simulink model "angle"  (R2024a)
settings: Solver=ode1  StartTime=0.0  StopTime=inf  FixedStep=0.01  RelTol=1e-3  EnableMultiTasking=on
libraries: arduinolib x4, slpidlib x1, arduinosensorlib x1, simulink_extras x1
settings Model: ExtModeTrigDuration=2  Creator=abane  LastModifiedBy=abane
settings SolverCC: AutoInsertRateTranBlk=on
settings OptimizationCC: EnhancedBackFolding=on  PassReuseOutputArgsAs=Individual arguments  ZeroExternalMemoryAtStartup=off  ZeroInternalMemoryAtStartup=off  MaxStackSize=64  OptimizeBlockOrder=speed  DifferentSizesBufferReuse=on  OptimizationCustomize=off  EfficientTunableParamExpr=on
settings DebuggingCC: ParameterTunabilityLossMsg=error
settings HardwareCC: ProdBitPerInt=16  ProdBitPerPointer=16  ProdBitPerSizeT=16  ProdBitPerPtrDiffT=16  ProdLargestAtomicFloat=None  ProdWordSize=8  ProdHWDeviceType=Atmel->AVR  UseEmbeddedCoderFeatures=off  UseSimulinkCoderFeatures=off
settings SFSimCC: MATLABDynamicMemAlloc=off
settings RTWCC: Description=Embedded Coder  SystemTargetFile=ert.tlc  HardwareBoard=Arduino Mega 2560  TemplateMakefile=ert_default_tmf  Toolchain=Arduino AVR  BuildConfiguration=Faster Runs
settings CodeAppCC: ForceParamTrailComments=on  IgnoreCustomStorageClasses=off  OperatorAnnotations=on  SimulinkDataObjDesc=on  SFDataObjDesc=on  InsertBlockDesc=on
settings ERTTargetCC: SupportContinuousTime=on  SupportNonInlinedSFcns=on  SupportVariableSizeSignals=on  ExtModeTransport=3  ExtModeStaticAlloc=on  ExtModeAutomaticAllocSize=off  ExtModeStaticAllocSize=2048  ExtModeMexFile=ext_xcp  ExtModeIntrfLevel=Level2 - Open

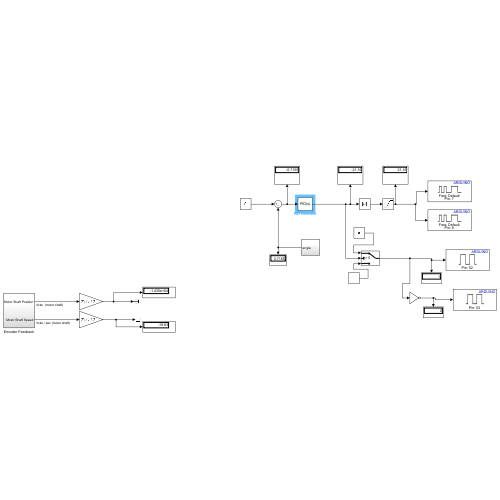
[thumbnail: Simulink's stored preview of the top-level diagram]
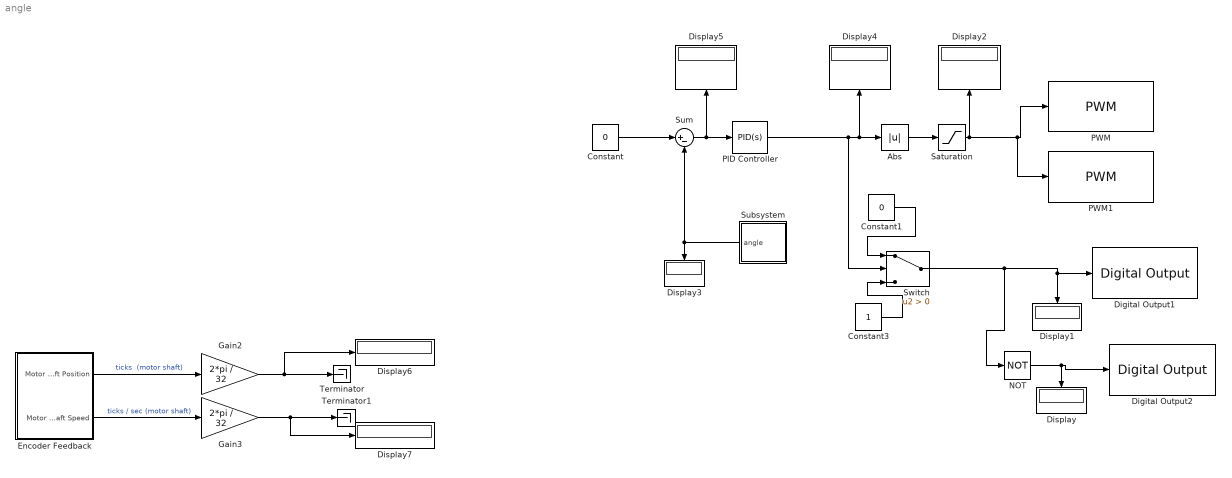
== system angle ==
  Abs : Abs  SaturateOnIntegerOverflow=off
  Constant : Constant  Value=0
  Constant1 : Constant  Value=0
  Constant3 : Constant
  Digital Output1 : arduinolib/Digital Output  pinNumber=52  Direction=output  blockPlatform=arduino
  Digital Output2 : arduinolib/Digital Output  pinNumber=53  Direction=output  blockPlatform=arduino
  Display{,1..7} (8 alike) : Display
  Encoder Feedback : Subsystem
  Gain2 : Gain  Gain=2*pi / 32
  Gain3 : Gain  Gain=2*pi / 32
  NOT : Logic  Operator=NOT  IconShape=distinctive  AllPortsSameDT=off  OutDataTypeStr=boolean
  PID Controller : slpidlib/PID Controller  Controller=PID  Form=Parallel  TimeDomain=Continuous-time  UseExternalTs=off  SampleTime=-1  IntegratorMethod=Forward Euler  FilterMethod=Forward Euler  ControllerParametersSource=internal  P=25  I=10  UseKiTs=off  D=0  UseExternalDerivativeSource=off  N=100  UseFilter=on  TunerSelectOption=Transfer Function Based (PID Tuner App)  InitialConditionSource=internal  InitialConditionForIntegrator=0  InitialConditionForFilter=0  DifferentiatorICPrevScaledInput=0  ExternalReset=none  TrackingMode=off  Kt=1  LimitOutput=off  SatLimitsSource=internal  UpperSaturationLimit=inf  LowerSaturationLimit=-inf  LinearizeAsGain=on  AntiWindupMode=none  Kb=1  LimitIntegrator=off  UpperIntegratorSaturationLimit=inf  LowerIntegratorSaturationLimit=-inf  POutMin=[]  POutMax=[]  IOutMin=[]  IOutMax=[]  DOutMin=[]  DOutMax=[]  NOutMin=[]  NOutMax=[]  SumOutMin=[]  SumOutMax=[]  SaturationOutMin=[]  SaturationOutMax=[]  PParamMin=[]  PParamMax=[]  IParamMin=[]  IParamMax=[]  DParamMin=[]  DParamMax=[]  NParamMin=[]  NParamMax=[]  KbParamMin=[]  KbParamMax=[]  KtParamMin=[]  KtParamMax=[]  KbOutMin=[]  KbOutMax=[]  KtOutMin=[]  KtOutMax=[]  IntegratorOutMin=[]  IntegratorOutMax=[]  FilterOutMin=[]  FilterOutMax=[]  SumI1OutMin=[]  SumI1OutMax=[]  SumI2OutMin=[]  SumI2OutMax=[]  SumI3OutMin=[]  SumI3OutMax=[]  SumI4OutMin=[]  SumI4OutMax=[]  SumDOutMin=[]  SumDOutMax=[]  DifferentiatorOutMin=[]  DifferentiatorOutMax=[]  FilterDiffOutCoefMin=[]  FilterDiffOutCoefMax=[]  ReciprocalOutMin=[]  ReciprocalOutMax=[]  SumDenOutMin=[]  SumDenOutMax=[]  SumNumOutMin=[]  SumNumOutMax=[]  DivideOutMin=[]  DivideOutMax=[]  UdiffTsProdOutMin=[]  UdiffTsProdOutMax=[]  NTsProdOutMin=[]  NTsProdOutMax=[]  UintegralTsProdOutMin=[]  UintegralTsProdOutMax=[]  UngainTsProdOutMin=[]  UngainTsProdOutMax=[]  ClampingZeroOutDataTypeStr=Inherit: Inherit via back propagation  ClampingZeroOutMin=[]  ClampingZeroOutMax=[]  FilterDenConstantOutDataTypeStr=Inherit: Inherit via back propagation  FilterDenConstantOutMin=[]  FilterDenConstantOutMax=[]  PCopyOutDataTypeStr=Inherit: Inherit via back propagation  PCopyOutMin=[]  PCopyOutMax=[]  NCopyOutDataTypeStr=Inherit: Inherit via back propagation  NCopyOutMin=[]  NCopyOutMax=[]  IntegratorContinuousStateAttributes=''  IntegratorStateMustResolveToSignalObject=off  IntegratorRTWStateStorageClass=Auto  FilterContinuousStateAttributes=''  FilterStateMustResolveToSignalObject=off  FilterRTWStateStorageClass=Auto  ParallelPVariant=InternalParameters  IdealPVariant=Disabled  IVariant=InternalParameters  DVariant=InternalParameters  IntegratorVariant=Continuous  SatVariant=Disabled  AWVariant=Passthrough  PCopyVariant=Disabled  TRVariant=Disabled  FdbkBlocksVariant=Forward  IdealPFdbkVariant=Disabled  SatFdbkVariant=Disabled  DerivativeFilterVariant=ContFilter  NVariant=InternalParameters  NCopyVariant=Disabled  FilterICVariant=InternalICsFilter  IntegratorICVariant=InternalICs  ExternalResetVariant=Disabled  TRSumVariant=Passthrough  SumFdbkVariant=Disabled  SumVariant=Sum_PID  TsampFilterVariant=InternalTs  TsampNgainVariant=Passthrough  TsampIntegralVariant=Disabled_SignalSpec  ExternalSaturationOutDataTypeStr=Inherit: Same as second input  DerivativeSourceVariant=ErrorSignal
  PWM : arduinolib/PWM  pinNumber=7  frequencyType=Default  desiredFrequency=490.2  achievableFrequency=490.2
  PWM1 : arduinolib/PWM  pinNumber=8  frequencyType=Default  desiredFrequency=490.2  achievableFrequency=490.2
  Saturation : Saturate  UpperLimit=255  LowerLimit=0
  Subsystem : Subsystem
  Sum : Sum  Inputs=|+-
  Switch : Switch  Criteria=u2 > Threshold  SaturateOnIntegerOverflow=off  InputSameDT=off
  Terminator : Terminator
  Terminator1 : Terminator
  wires:
  Sum/1 -> PID Controller/1, Display5/1
  Saturation/1 -> PWM1/1, PWM/1, Display2/1
  Subsystem/1(angle) -> Display3/1, Sum/2
  Constant/1 -> Sum/1
  Constant1/1 -> Switch/1
  Constant3/1 -> Switch/3
  Switch/1 -> NOT/1, Digital Output1/1, Display1/1
  PID Controller/1 -> Display4/1, Abs/1, Switch/2
  NOT/1 -> Digital Output2/1, Display/1
  Abs/1 -> Saturation/1
  Encoder Feedback/2(Motor Shaft Speed) -> Gain3/1  "ticks / sec (motor shaft)"
  Gain3/1 -> Display7/1, Terminator1/1
  Encoder Feedback/1(Motor Shaft Position) -> Gain2/1  "ticks  (motor shaft)"
  Gain2/1 -> Display6/1, Terminator/1

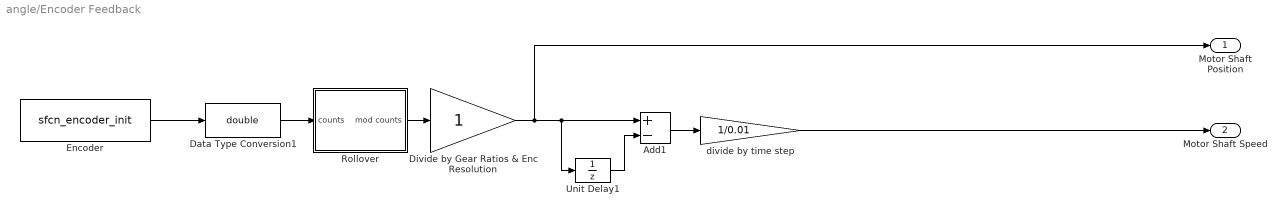
== system angle/Encoder Feedback ==
  Add1 : Sum  Inputs=+-
  Data Type Conversion1 : DataTypeConversion  OutDataTypeStr=double  SaturateOnIntegerOverflow=off  RndMeth=Floor
  Divide by Gear Ratios & Enc Resolution : Gain
  Encoder : S-Function  InitFcn=try, set_param(gcb,'FunctionName','sfcn_encoder_init'), end  FunctionName=sfcn_encoder_init  Parameters=uint8(0),uint8(3),uint8(1)  SFunctionModules=sfcn_encoder_init_wrapper.c  SFunctionDeploymentMode=off  EnableBusSupport=off  mask(S-Function Builder){}
      mask init:
      | val = [[.9  0.75 0.75 1 1 .9 .9 1]',[1 1 0.75 0.75 .9 .9 1 .9]'];try , sys = get_param(gcb,'SfunBuilderFcnName');if isempty(sys), sys = get_param(gcb,'FunctionName'); end,catch, sys = get_param(gcb,'FunctionName'); end
      settings: CopyFcn=set_param(gcbh,'LinkStatus','none')  PreSaveFcn=try, set_param(gcb,'FunctionName','sfcn_encoder_init'), end  OpenFcn=sfunctionwizard(gcbh)
      mask Display: plot(val(:,1),val(:,2)),disp(sys), port_label('output',1,'pos')
  Rollover : Subsystem
  Unit Delay1 : UnitDelay  SampleTime=-1  HasFrameUpgradeWarning=on
  divide by time step : Gain  Gain=1/0.01
  Motor Shaft Position : Outport
  Motor Shaft Speed : Outport  Port=2
  wires:
  Encoder/1 -> Data Type Conversion1/1
  Unit Delay1/1 -> Add1/2
  Data Type Conversion1/1 -> Rollover/1(counts)
  divide by time step/1 -> Motor Shaft Speed/1
  Add1/1 -> divide by time step/1
  Rollover/1(" mod counts") -> Divide by Gear Ratios & Enc Resolution/1
  Divide by Gear Ratios & Enc Resolution/1 -> Motor Shaft Position/1, Add1/1, Unit Delay1/1

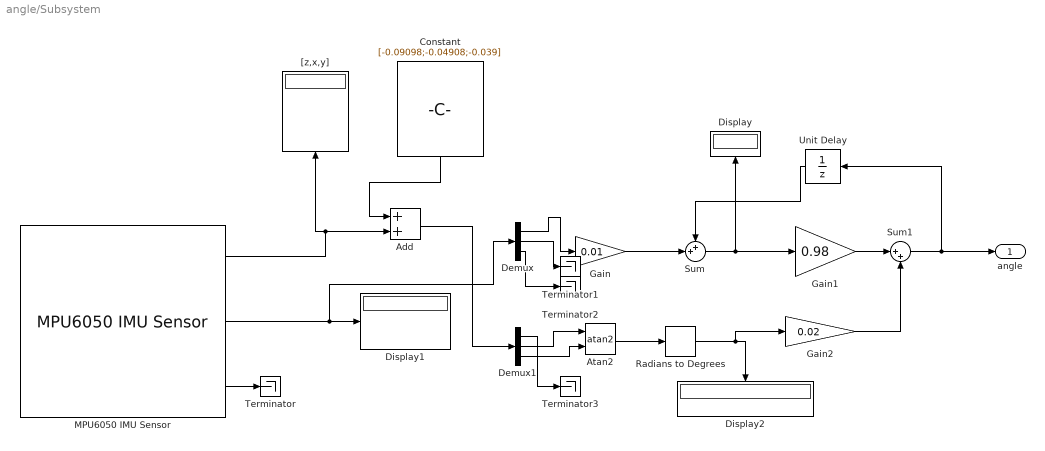
== system angle/Subsystem ==
  Add : Sum
  Atan2 : Trigonometry  Operator=atan2
  Constant : Constant  Value=[-0.09098;-0.04908;-0.039]  VectorParams1D=off
  Demux : Demux  Outputs=3
  Demux1 : Demux  Outputs=3
  Display : Display
  Display1 : Display
  Display2 : Display
  Gain : Gain  Gain=0.01
  Gain1 : Gain  Gain=0.98
  Gain2 : Gain  Gain=0.02
  MPU6050 IMU Sensor : arduinosensorlib/MPU6050 IMU Sensor  I2CModule=0  SlaveAddress=0x68  Accel=on  AngularRate=on  Temperature=off  Status=on  Timestamp=off  EulerAngles=off  Quat=off  AccelRange=2G  GyroRange=250 dps  DmpOdr=200 Hz  Dlpf=Accelerometer: 184Hz, Gyroscope: 188Hz  spf=1  SampleTime=-1  QueueSizeFactor=1
  Radians to Degrees : simulink_extras/Transformations/Radians to Degrees
  Sum : Sum  Inputs=++|
  Sum1 : Sum  Inputs=|++
  Terminator{,1..3} (4 alike) : Terminator
  Unit Delay : UnitDelay  SampleTime=-1  HasFrameUpgradeWarning=on
  "[z,x,y]" : Display
  angle : Outport
  wires:
  MPU6050 IMU Sensor/1 -> Add/2, "[z,x,y]"/1
  Demux1/1 -> Terminator3/1
  Sum/1 -> Gain1/1, Display/1
  MPU6050 IMU Sensor/2 -> Demux/1, Display1/1
  Gain/1 -> Sum/2
  Add/1 -> Demux1/1
  Constant/1 -> Add/1
  Atan2/1 -> Radians to Degrees/1
  Gain1/1 -> Sum1/1
  Demux/3 -> Terminator2/1
  Demux1/2 -> Atan2/1
  Demux1/3 -> Atan2/2
  Gain2/1 -> Sum1/2
  Radians to Degrees/1 -> Gain2/1, Display2/1
  MPU6050 IMU Sensor/3 -> Terminator/1
  Sum1/1 -> angle/1, Unit Delay/1
  Demux/1 -> Gain/1
  Unit Delay/1 -> Sum/1
  Demux/2 -> Terminator1/1

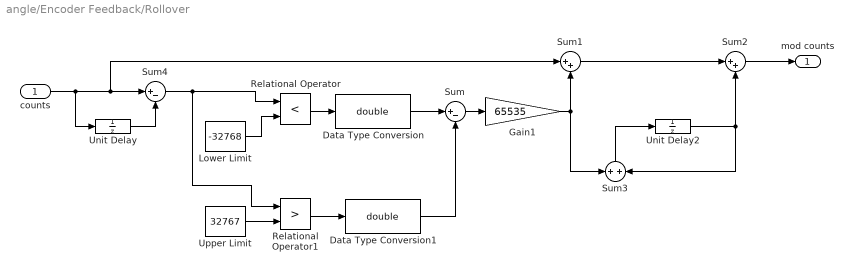
== system angle/Encoder Feedback/Rollover ==
  counts : Inport
  " Lower Limit" : Constant  Value=-32768
  " Upper Limit" : Constant  Value=32767
  Data Type Conversion : DataTypeConversion  OutDataTypeStr=double  SaturateOnIntegerOverflow=off
  Data Type Conversion1 : DataTypeConversion  OutDataTypeStr=double  SaturateOnIntegerOverflow=off
  Gain1 : Gain  Gain=65535
  Relational Operator : RelationalOperator  Operator=<  OutDataTypeStr=boolean  InputSameDT=off
  Relational Operator1 : RelationalOperator  Operator=>  OutDataTypeStr=boolean  InputSameDT=off
  Sum : Sum  Inputs=|+-
  Sum1 : Sum  Inputs=|++  OutDataTypeStr=double
  Sum2 : Sum  Inputs=|++
  Sum3 : Sum
  Sum4 : Sum  Inputs=|+-
  Unit Delay : UnitDelay  SampleTime=-1  HasFrameUpgradeWarning=on
  Unit Delay2 : UnitDelay  SampleTime=-1  HasFrameUpgradeWarning=on
  " mod counts" : Outport
  wires:
  counts/1 -> Unit Delay/1, Sum1/1, Sum4/1
  Sum2/1 -> " mod counts"/1
  Unit Delay/1 -> Sum4/2
  Data Type Conversion/1 -> Sum/1
  Sum3/1 -> Unit Delay2/1
  Data Type Conversion1/1 -> Sum/2
  Sum/1 -> Gain1/1
  Gain1/1 -> Sum1/2, Sum3/1
  Relational Operator1/1 -> Data Type Conversion1/1
  Sum1/1 -> Sum2/1
  Relational Operator/1 -> Data Type Conversion/1
  " Upper Limit"/1 -> Relational Operator1/2
  Unit Delay2/1 -> Sum3/2, Sum2/2
  " Lower Limit"/1 -> Relational Operator/2
  Sum4/1 -> Relational Operator/1, Relational Operator1/1
